simulink model "sampleModel1829_sub_sub"  (R2023a)
settings: Solver=VariableStepAuto  StartTime=0.0  StopTime=10.0  RelTol=1e-3
libraries: simulink x2, hdlsllib x2
settings Model: Creator=user1  LastModifiedBy=user1

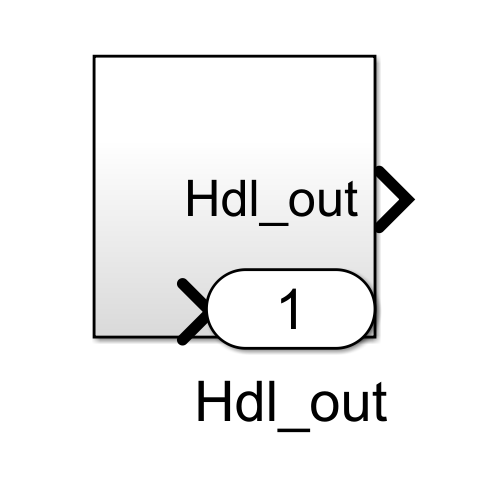
[thumbnail: Simulink's stored preview of the top-level diagram]
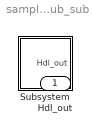
== system sampleModel1829_sub_sub ==
  Subsystem : Subsystem
  Hdl_out : Outport  OutDataTypeStr=uint8

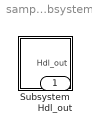
== system sampleModel1829_sub_sub/Subsystem ==
  Subsystem : Subsystem
  Hdl_out : Outport  OutDataTypeStr=uint8

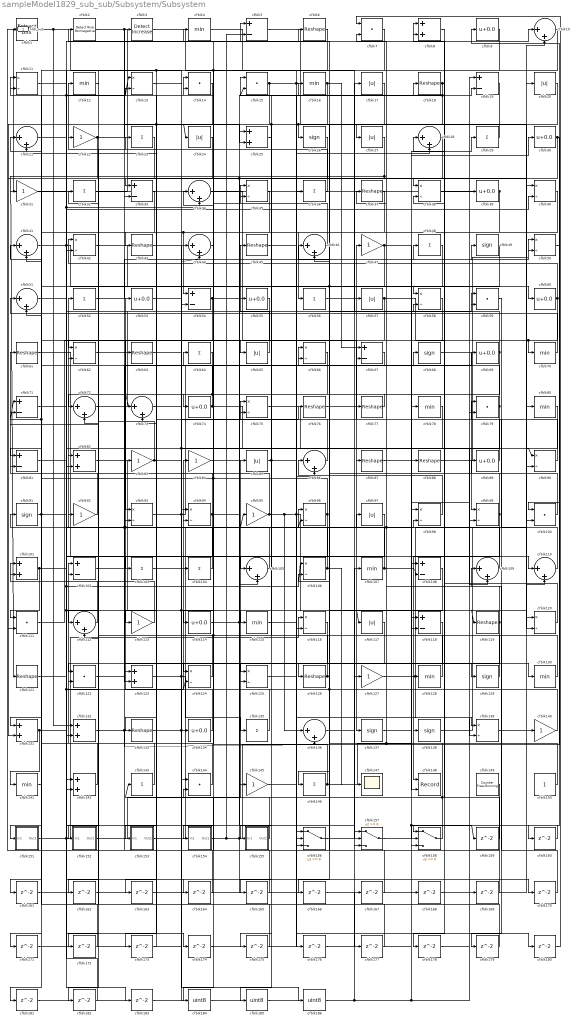
== system sampleModel1829_sub_sub/Subsystem/Subsystem ==
  cfblk1 : simulink/Logic and Bit Operations/Extract Bits  bitsToExtract=Upper half  numBits=8  bitIdxRange=[0 7]  outScalingMode=Preserve fixed-point scaling
      settings: LibrarySourceBlock=|
      | hdlsllib/Logic and Bit
      | Operations/Extract Bits
  cfblk{10,21,28,34,41,44,46,51,72..73,86,105,109..110,112,136} (16 alike) : Sum  Inputs=|++  OutDataTypeStr=uint8
  cfblk{7,14..15,59,79,100,111,122,144} (9 alike) : DotProduct  OutDataTypeStr=uint8
  cfblk{8,25,82,101,123,131..132,142} (8 alike) : Sum  OutDataTypeStr=uint8
  cfblk{5,19,33,54,67,71,81,102,108,118} (10 alike) : Sum  Inputs=+-  OutDataTypeStr=uint8
  cfblk{23,29,32,36,48,52,56,64,103..104,135,143,146} (13 alike) : Sum  Inputs=+  OutDataTypeStr=uint8
  cfblk{11,13,35,38,40,42,50,58,62,66,75,90,93..94,96,98..99,106,116,120,124..125,139} (23 alike) : Product  Inputs=*/  OutDataTypeStr=uint8  RndMeth=Zero  SaturateOnIntegerOverflow=on
  cfblk{4,12,16,70,78,80,107,115,128,130,141} (11 alike) : MinMax  OutDataTypeStr=uint8
  cfblk{22,31,47,83..84,92,95,113,127,140,145} (11 alike) : Gain  OutDataTypeStr=uint8
  cfblk{9,30,39,53,55,60,69,74,89,114,134} (11 alike) : Bias  Bias=0.0  SaturateOnIntegerOverflow=off
  cfblk{17,20,24,27,57,65,85,97,117} (9 alike) : Abs  OutDataTypeStr=uint8  SaturateOnIntegerOverflow=off
  cfblk{6,18,37,43,45,61,63,76..77,87..88,119,121,126,133} (15 alike) : Reshape
  cfblk{26,49,68,91,129,137..138} (7 alike) : Signum
  cfblk147 : Scope
  cfblk148 : Record  FileSettingsInternal="{\"entries\":[{\"content\":{\"excelSettings\":{\"content\":{},\"type\":\"Streamout.ExcelSettings\"}},\"type\":\"Streamout.FileSettingStorage\",\"uuid\":\"\"}],\"packageUris\":[\"http:\\/\\/schema.mathworks.com\\/mf0\\/streamout_blocks\\/R2020a\"],\"version\":\"1.0\"}"  Layout=[1 1]  SignalsInternal="{\"entries\":[{\"content\":{\"signals\":[{\"content\":{\"blockPath\":[],\"dimensions\":[1],\"domain\":\"\",\"lineColor\":\"#a2142f\",\"plots\":[1],\"port\":1,\"signalID\":43963,\"signalName\":\"cfblk99\"},\"type\":\"RecordBlkView.Signal\",\"uuid\":\"\"},{\"content\":{\"blockPath\":[],\"dimensions\":[1],\"domain\":\"\",\"lineColor\":\"#139fff\",\"plots\":[1],\"port\":2,\"signalID\":43966,\"signalName\":\"cfblk74\"},\"type\":\"RecordBlkView.Signal\",\"uuid\":\"\"}]},\"type\":\"RecordBlkView.InputSignals\",\"uuid\":\"\"}],\"packageUris\":[\"http:\\/\\/schema.mathworks.com\\/mf0\\/streamout_blocks\\/R2020a\"],\"version\":\"1.0\"}"  VisualizationBindings="{\"xyplotplugin\":{\"info\":[{\"series\":[{\"bindingParametersList\":[{\"parameter\":\"X-Axis\",\"signalID\":43963,\"signalName\":\"cfblk99\"},{\"parameter\":\"Y-Axis\",\"signalID\":43966,\"signalName\":\"cfblk74\"}],\"seriesID\":241}],\"subplotID\":1}]}}"  CompatibilityTag=XY  st=-1
  cfblk149 : hdlsllib/Sources/Counter Free-Running  NumBits=16  tsamp=-1
  cfblk150 : Constant  OutDataTypeStr=uint8  SampleTime=-1
  cfblk151 : Subsystem
      settings: LibrarySourceBlock=|
      | hdlsllib/Ports &
      | Subsystems/Subsystem
  cfblk152 : Subsystem
      settings: LibrarySourceBlock=|
      | hdlsllib/Ports &
      | Subsystems/Subsystem
  cfblk153 : Subsystem
      settings: LibrarySourceBlock=|
      | hdlsllib/Ports &
      | Subsystems/Subsystem
  cfblk154 : Subsystem
      settings: LibrarySourceBlock=|
      | hdlsllib/Ports &
      | Subsystems/Subsystem
  cfblk155 : Subsystem
      settings: LibrarySourceBlock=|
      | hdlsllib/Ports &
      | Subsystems/Subsystem
  cfblk156 : Switch  OutDataTypeStr=uint8  SaturateOnIntegerOverflow=off  InputSameDT=off
  cfblk157 : Switch  OutDataTypeStr=uint8  SaturateOnIntegerOverflow=off  InputSameDT=off
  cfblk158 : Switch  OutDataTypeStr=uint8  SaturateOnIntegerOverflow=off  InputSameDT=off
  cfblk{159..183} (25 alike) : Delay  SampleTime=1
  cfblk184 : DataTypeConversion  OutDataTypeStr=uint8  SaturateOnIntegerOverflow=off  RndMeth=Floor
  cfblk185 : DataTypeConversion  OutDataTypeStr=uint8  SaturateOnIntegerOverflow=off  RndMeth=Floor
  cfblk186 : DataTypeConversion  OutDataTypeStr=uint8  SaturateOnIntegerOverflow=off  RndMeth=Floor
  cfblk2 : hdlsllib/Logic and Bit Operations/Detect Rise Nonnegative  vinit=0  OutDataTypeStr=uint8
  cfblk3 : simulink/Logic and Bit Operations/Detect Increase  vinit=0.0  OutDataTypeStr=uint8
      settings: LibrarySourceBlock=|
      | hdlsllib/Logic and Bit
      | Operations/Detect
      | Increase
  Hdl_out : Outport  OutDataTypeStr=uint8
  wires:
  cfblk186/1 -> cfblk118/2
  cfblk185/1 -> cfblk118/1
  cfblk184/1 -> cfblk169/1, cfblk168/1, cfblk167/1
  cfblk183/1 -> cfblk79/2
  cfblk182/1 -> cfblk142/1
  cfblk97/1 -> cfblk182/1
  cfblk181/1 -> cfblk54/2
  cfblk180/1 -> cfblk7/1
  cfblk179/1 -> cfblk11/2
  cfblk59/1 -> cfblk179/1
  cfblk178/1 -> cfblk19/1
  cfblk49/1 -> cfblk178/1
  cfblk177/1 -> cfblk102/2
  cfblk136/1 -> cfblk177/1
  cfblk176/1 -> cfblk158/3
  cfblk145/1 -> cfblk176/1
  cfblk175/1 -> cfblk94/1
  cfblk117/1 -> cfblk175/1
  cfblk174/1 -> cfblk156/1
  cfblk173/1 -> cfblk13/2
  cfblk64/1 -> cfblk173/1
  cfblk172/1 -> cfblk51/2
  cfblk12/1 -> cfblk172/1
  cfblk171/1 -> cfblk44/1
  cfblk14/1 -> cfblk171/1
  cfblk170/1 -> cfblk109/1
  cfblk31/1 -> cfblk170/1
  cfblk169/1 -> cfblk46/2
  cfblk168/1 -> cfblk40/1
  cfblk167/1 -> cfblk144/2
  cfblk166/1 -> cfblk98/1
  cfblk17/1 -> cfblk166/1
  cfblk165/1 -> cfblk122/2
  cfblk25/1 -> cfblk165/1
  cfblk164/1 -> cfblk123/1
  cfblk21/1 -> cfblk164/1
  cfblk163/1 -> cfblk86/2
  cfblk58/1 -> cfblk163/1
  cfblk162/1 -> cfblk110/2
  cfblk116/1 -> cfblk162/1
  cfblk161/1 -> cfblk75/2
  cfblk160/1 -> cfblk158/2
  cfblk159/1 -> cfblk38/2
  cfblk126/1 -> cfblk82/1, cfblk106/2
  cfblk108/1 -> cfblk146/1
  cfblk5/1 -> cfblk100/2
  cfblk137/1 -> cfblk59/1
  cfblk6/1 -> cfblk43/1, cfblk152/1(In1)
  cfblk139/1 -> cfblk140/1
  cfblk131/1 -> cfblk141/1, cfblk59/2
  cfblk16/1 -> cfblk105/1, cfblk112/1, cfblk67/1
  cfblk115/1 -> cfblk139/1
  cfblk110/1 -> cfblk79/1
  cfblk56/1 -> cfblk57/1
  cfblk96/1 -> cfblk4/1, cfblk41/2, cfblk185/1
  cfblk132/1 -> cfblk69/1, cfblk96/2, cfblk136/2
  cfblk107/1 -> cfblk108/2, cfblk14/2
  cfblk54/1 -> cfblk83/1, cfblk18/1
  cfblk62/1 -> cfblk130/1
  cfblk67/1 -> cfblk66/2
  cfblk155/1(Out1) -> cfblk145/1
  cfblk4/1 -> cfblk36/1
  cfblk43/1 -> cfblk60/1
  cfblk158/1 -> cfblk143/1, cfblk2/1
  cfblk146/1 -> cfblk34/1, cfblk78/1
  cfblk75/1 -> cfblk109/2
  cfblk78/1 -> cfblk155/1(In1)
  cfblk69/1 -> cfblk157/2, cfblk6/1
  cfblk3/1 -> cfblk127/1
  cfblk76/1 -> cfblk47/1
  cfblk150/1 -> cfblk37/1, cfblk16/1
  cfblk60/1 -> cfblk70/1, cfblk73/2, cfblk42/1
  cfblk47/1 -> cfblk99/2, cfblk112/2
  cfblk38/1 -> cfblk39/1
  cfblk42/1 -> cfblk108/1
  cfblk8/1 -> cfblk58/1
  cfblk124/1 -> cfblk63/1
  cfblk79/1 -> cfblk46/1, cfblk82/2
  cfblk103/1 -> cfblk129/1
  cfblk10/1 -> cfblk31/1
  cfblk114/1 -> cfblk25/1, cfblk157/3
  cfblk109/1 -> cfblk35/2, cfblk7/2
  cfblk125/1 -> cfblk156/2
  cfblk86/1 -> cfblk75/1
  cfblk30/1 -> cfblk160/1, cfblk161/1
  cfblk15/1 -> cfblk120/1, cfblk180/1, cfblk42/2
  cfblk101/1 -> cfblk93/2, cfblk95/1, cfblk111/1
  cfblk72/1 -> cfblk17/1
  cfblk63/1 -> cfblk49/1
  cfblk94/1 -> cfblk41/1, cfblk71/1, cfblk142/2, cfblk105/2
  cfblk89/1 -> cfblk21/2
  cfblk19/1 -> cfblk27/1
  cfblk106/1 -> cfblk81/2, cfblk147/1
  cfblk91/1 -> cfblk151/1(In1), cfblk183/1
  cfblk122/1 -> cfblk66/1
  cfblk104/1 -> cfblk22/1
  cfblk102/1 -> cfblk98/2
  cfblk33/1 -> cfblk81/1
  cfblk28/1 -> cfblk125/1
  cfblk71/1 -> cfblk55/1
  cfblk13/1 -> cfblk104/1
  cfblk85/1 -> cfblk15/1, cfblk28/2
  cfblk24/1 -> cfblk72/2
  cfblk128/1 -> cfblk35/1
  cfblk55/1 -> cfblk93/1
  cfblk127/1 -> cfblk10/2, cfblk139/2
  cfblk121/1 -> cfblk10/1, cfblk34/2, cfblk106/1
  cfblk7/1 -> cfblk123/2
  cfblk130/1 -> cfblk8/2
  cfblk129/1 -> cfblk94/2, cfblk71/2
  cfblk11/1 -> cfblk103/1
  cfblk87/1 -> cfblk29/1
  cfblk82/1 -> cfblk138/1
  cfblk120/1 -> cfblk28/1
  cfblk92/1 -> cfblk61/1
  cfblk52/1 -> cfblk50/2
  cfblk84/1 -> cfblk48/1
  cfblk73/1 -> cfblk119/1, cfblk186/1
  cfblk113/1 -> cfblk92/1
  cfblk65/1 -> cfblk45/1
  cfblk98/1 -> cfblk86/1
  cfblk119/1 -> cfblk122/1, cfblk77/1
  cfblk100/1 -> cfblk64/1
  cfblk90/1 -> cfblk8/1
  cfblk142/1 -> cfblk91/1
  cfblk74/1 -> cfblk21/1, cfblk73/1, cfblk148/2
  cfblk37/1 -> cfblk56/1
  cfblk66/1 -> cfblk114/1
  cfblk133/1 -> cfblk134/1, cfblk76/1
  cfblk39/1 -> cfblk158/1, Hdl_out/1
  cfblk22/1 -> cfblk3/1, cfblk131/2
  cfblk99/1 -> cfblk148/1, cfblk89/1
  cfblk149/1 -> cfblk1/1
  cfblk29/1 -> cfblk26/1, cfblk24/1
  cfblk51/1 -> cfblk13/1, cfblk5/1
  cfblk77/1 -> cfblk72/1
  cfblk141/1 -> cfblk101/2
  cfblk156/1 -> cfblk107/1
  cfblk9/1 -> cfblk74/1, cfblk132/2
  cfblk45/1 -> cfblk116/2
  cfblk112/1 -> cfblk101/1
  cfblk53/1 -> cfblk110/1
  cfblk48/1 -> cfblk126/1, cfblk181/1
  cfblk123/1 -> cfblk135/1, cfblk67/2
  cfblk138/1 -> cfblk20/1
  cfblk140/1 -> cfblk14/1, cfblk96/1
  cfblk118/1 -> cfblk184/1
  cfblk144/1 -> cfblk32/1
  cfblk50/1 -> cfblk100/1
  cfblk35/1 -> cfblk113/1
  cfblk44/1 -> cfblk154/1(In1)
  cfblk80/1 -> cfblk90/2
  cfblk18/1 -> cfblk133/1, cfblk111/2, cfblk15/2, cfblk128/1
  cfblk81/1 -> cfblk117/1, cfblk174/1
  cfblk70/1 -> cfblk51/1
  cfblk157/1 -> cfblk30/1, cfblk159/1
  cfblk135/1 -> cfblk53/1
  cfblk95/1 -> cfblk120/2, cfblk19/2, cfblk136/1, cfblk23/1
  cfblk26/1 -> cfblk33/2
  cfblk83/1 -> cfblk90/1, cfblk44/2, cfblk62/2
  cfblk41/1 -> cfblk88/1, cfblk156/3
  cfblk1/1 -> cfblk144/1, cfblk132/1
  cfblk134/1 -> cfblk84/1
  cfblk40/1 -> cfblk54/1, cfblk153/1(In1)
  cfblk151/1(Out1) -> cfblk40/2, cfblk124/2, cfblk116/1
  cfblk153/1(Out1) -> cfblk97/1
  cfblk61/1 -> cfblk157/1
  cfblk20/1 -> cfblk62/1
  cfblk2/1 -> cfblk80/1, cfblk25/2
  cfblk34/1 -> cfblk87/1
  cfblk105/1 -> cfblk52/1
  cfblk152/1(Out1) -> cfblk85/1
  cfblk154/1(Out1) -> cfblk9/1, cfblk58/2, cfblk5/2
  cfblk68/1 -> cfblk99/1
  cfblk57/1 -> cfblk137/1, cfblk131/1
  cfblk36/1 -> cfblk12/1
  cfblk111/1 -> cfblk65/1
  cfblk143/1 -> cfblk102/1
  cfblk23/1 -> cfblk33/1
  cfblk88/1 -> cfblk50/1
  cfblk46/1 -> cfblk11/1
  cfblk27/1 -> cfblk125/2, cfblk124/1, cfblk121/1
  cfblk93/1 -> cfblk68/1, cfblk115/1
  cfblk32/1 -> cfblk38/1

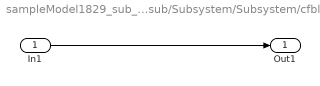
== system sampleModel1829_sub_sub/Subsystem/Subsystem/cfblk151 ==
  In1 : Inport
  Out1 : Outport
  wires:
  In1/1 -> Out1/1

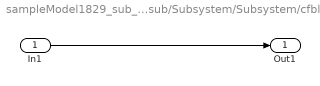
== system sampleModel1829_sub_sub/Subsystem/Subsystem/cfblk152 ==
  In1 : Inport
  Out1 : Outport
  wires:
  In1/1 -> Out1/1

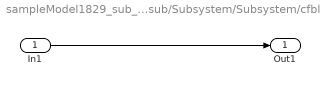
== system sampleModel1829_sub_sub/Subsystem/Subsystem/cfblk153 ==
  In1 : Inport
  Out1 : Outport
  wires:
  In1/1 -> Out1/1

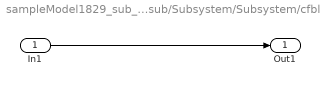
== system sampleModel1829_sub_sub/Subsystem/Subsystem/cfblk154 ==
  In1 : Inport
  Out1 : Outport
  wires:
  In1/1 -> Out1/1

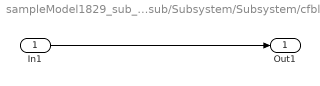
== system sampleModel1829_sub_sub/Subsystem/Subsystem/cfblk155 ==
  In1 : Inport
  Out1 : Outport
  wires:
  In1/1 -> Out1/1
